simulink model "untitled"  (R2020a)
settings: Solver=VariableStepAuto  StartTime=0.0  StopTime=100  RelTol=1e-3
settings Model: Creator=rezoa  LastModifiedBy=rezoa

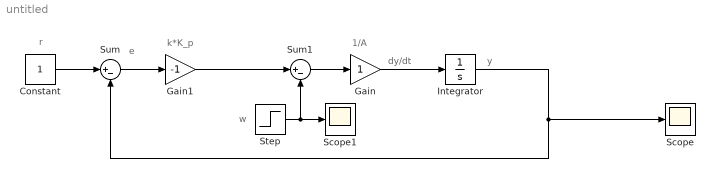
== system untitled ==
  note: w
  note: e
  note: r
  note: k*K_p
  note: 1/A
  note: dy/dt
  note: y
  Constant : Constant
  Gain : Gain
  Gain1 : Gain  Gain=-1
  Integrator : Integrator  InitialCondition=0.5
  Scope : Scope
  Scope1 : Scope
  Step : Step  Time=10  After=0.1  SampleTime=0
  Sum : Sum  Inputs=|+-
  Sum1 : Sum  Inputs=|+-
  wires:
  Sum/1 -> Gain1/1
  Step/1 -> Sum1/2, Scope1/1
  Integrator/1 -> Scope/1, Sum/2
  Sum1/1 -> Gain/1
  Gain/1 -> Integrator/1
  Gain1/1 -> Sum1/1
  Constant/1 -> Sum/1
